simulink model "Aplicatia_2"  (R2017b)
settings: Solver=ode4  StartTime=0.0  StopTime=6  FixedStep=0.01  RelTol=1e-3
libraries: simulink x4
settings Model: Creator=tutuc  LastModifiedBy=tutuc

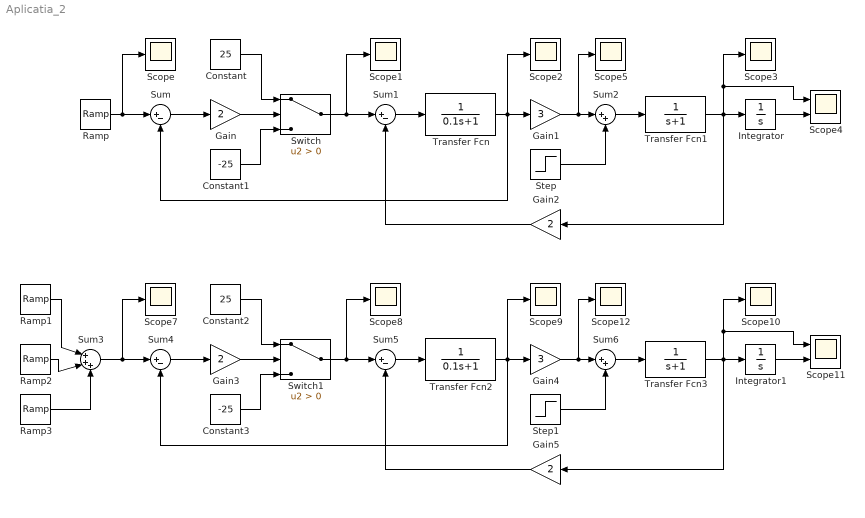
== system Aplicatia_2 ==
  Constant : Constant  Value=25
  Constant1 : Constant  Value=-25
  Constant2 : Constant  Value=25
  Constant3 : Constant  Value=-25
  Gain{,2..3,5} (4 alike) : Gain  Gain=2
  Gain1 : Gain  Gain=3
  Gain4 : Gain  Gain=3
  Integrator : Integrator
  Integrator1 : Integrator
  Ramp : simulink/Sources/Ramp  slope=2  start=0  X0=0
  Ramp1 : simulink/Sources/Ramp  slope=4  start=0  X0=0
  Ramp2 : simulink/Sources/Ramp  slope=-4  start=2  X0=0
  Ramp3 : simulink/Sources/Ramp  slope=-3  start=4  X0=0
  Scope{,1..3,5,7..10,12} (10 alike) : Scope
  Scope11 : Scope  NumInputPorts=2
  Scope4 : Scope  NumInputPorts=2
  Step : Step  Time=2.5  After=15  SampleTime=0
  Step1 : Step  Time=2.5  After=15  SampleTime=0
  Sum{,1,4..5} (4 alike) : Sum  Inputs=|+-
  Sum2 : Sum  Inputs=|++
  Sum3 : Sum  Inputs=|+++
  Sum6 : Sum  Inputs=|++
  Switch : Switch  Criteria=u2 > Threshold
  Switch1 : Switch  Criteria=u2 > Threshold
  Transfer Fcn : TransferFcn  Denominator=[0.1 1]
  Transfer Fcn1 : TransferFcn  Denominator=[1 1]
  Transfer Fcn2 : TransferFcn  Denominator=[0.1 1]
  Transfer Fcn3 : TransferFcn  Denominator=[1 1]
  wires:
  Ramp/1 -> Scope/1, Sum/1
  Sum/1 -> Gain/1
  Gain/1 -> Switch/2
  Constant1/1 -> Switch/3
  Constant/1 -> Switch/1
  Switch/1 -> Scope1/1, Sum1/1
  Sum1/1 -> Transfer Fcn/1
  Transfer Fcn/1 -> Sum/2, Scope2/1, Gain1/1
  Gain1/1 -> Scope5/1, Sum2/1
  Step/1 -> Sum2/2
  Sum2/1 -> Transfer Fcn1/1
  Transfer Fcn1/1 -> Gain2/1, Scope4/1, Scope3/1, Integrator/1
  Integrator/1 -> Scope4/2
  Gain2/1 -> Sum1/2
  Ramp2/1 -> Sum3/2
  Ramp1/1 -> Sum3/1
  Ramp3/1 -> Sum3/3
  Gain5/1 -> Sum5/2
  Integrator1/1 -> Scope11/2
  Transfer Fcn3/1 -> Integrator1/1, Scope10/1, Scope11/1, Gain5/1
  Sum6/1 -> Transfer Fcn3/1
  Step1/1 -> Sum6/2
  Gain4/1 -> Sum6/1, Scope12/1
  Transfer Fcn2/1 -> Gain4/1, Scope9/1, Sum4/2
  Sum5/1 -> Transfer Fcn2/1
  Switch1/1 -> Sum5/1, Scope8/1
  Constant2/1 -> Switch1/1
  Constant3/1 -> Switch1/3
  Gain3/1 -> Switch1/2
  Sum4/1 -> Gain3/1
  Sum3/1 -> Sum4/1, Scope7/1
